simulink model "blocos"  (R2013a)
settings: Solver=ode45  StartTime=0.0  StopTime=10.0  RelTol=1e-3
settings Model: Creator=Guilherme  LastModifiedBy=Guilherme

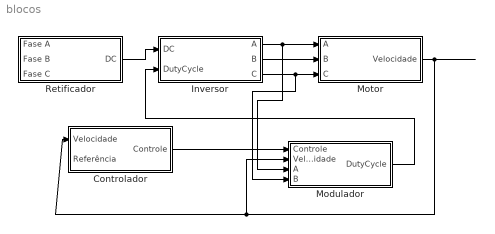
== system blocos ==
  Controlador : Subsystem
  Inversor : Subsystem
  Modulador : Subsystem
  Motor : Subsystem
  Retificador : Subsystem
  wires:
  Retificador/1(DC) -> Inversor/1(DC)
  Inversor/1(A) -> Modulador/3(A), Motor/1(A)
  Inversor/2(B) -> Motor/2(B)
  Inversor/3(C) -> Modulador/4(B), Motor/3(C)
  Motor/1(Velocidade) -> Controlador/1(Velocidade), Modulador/2(Velocidade)
  ? -> Controlador/2(Referência)
  ? -> Retificador/1(Fase A)
  ? -> Retificador/2(Fase B)
  ? -> Retificador/3(Fase C)
  Modulador/1(DutyCycle) -> Inversor/2(DutyCycle)
  Controlador/1(Controle) -> Modulador/1(Controle)

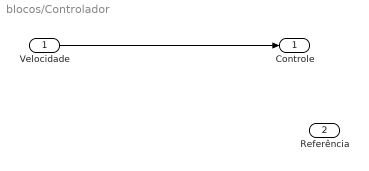
== system blocos/Controlador ==
  Velocidade : Inport
  Referência : Inport  Port=2
  Controle : Outport
  wires:
  Velocidade/1 -> Controle/1

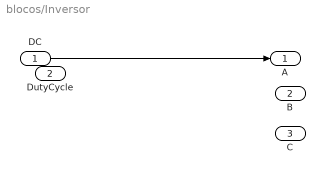
== system blocos/Inversor ==
  DC : Inport
  DutyCycle : Inport  Port=2
  A : Outport
  B : Outport  Port=2
  C : Outport  Port=3
  wires:
  DC/1 -> A/1

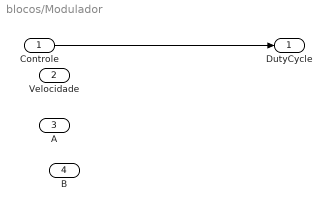
== system blocos/Modulador ==
  Controle : Inport
  Velocidade : Inport  Port=2
  A : Inport  Port=3
  B : Inport  Port=4
  DutyCycle : Outport
  wires:
  Controle/1 -> DutyCycle/1

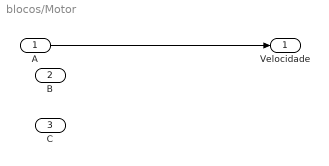
== system blocos/Motor ==
  A : Inport
  B : Inport  Port=2
  C : Inport  Port=3
  Velocidade : Outport
  wires:
  A/1 -> Velocidade/1

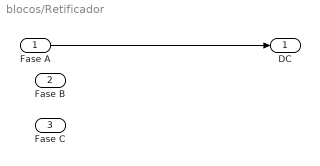
== system blocos/Retificador ==
  Fase A : Inport
  Fase B : Inport  Port=2
  Fase C : Inport  Port=3
  DC : Outport
  wires:
  Fase A/1 -> DC/1
